simulink model "PMSM_controller"  (R2021b)
settings: Solver=VariableStepAuto  StartTime=0.0  StopTime=1  RelTol=1e-3
values from neighbouring files (symbols this model uses):
  J = 0.2    [Para_Trial.m]
  Tmax = 27    [Para_Trial.m]
  Ts = 2e-6    (= 2e-06)    [Para_Trial.m]
  Tsc = 5e-5    (= 5e-05)    [Para_Trial.m]
libraries: eePmsmFieldOrientedControl x1
settings Model: Creator=Patron  LastModifiedBy=Patron
settings SolverCC: ZeroCrossAlgorithm=Adaptive
settings DataIOCC: SaveOutput=off  SaveTime=off
settings DebuggingCC: IgnoredZcDiagnostic=none

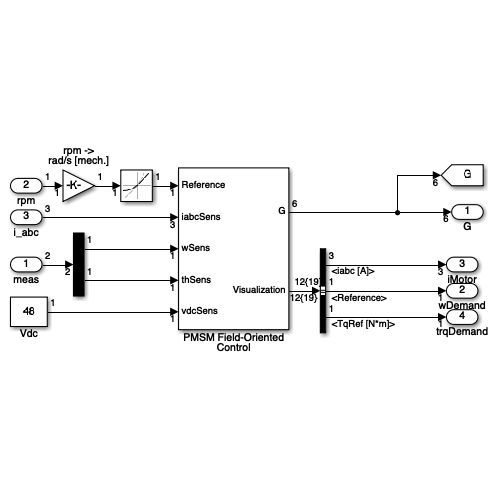
[thumbnail: Simulink's stored preview of the top-level diagram]
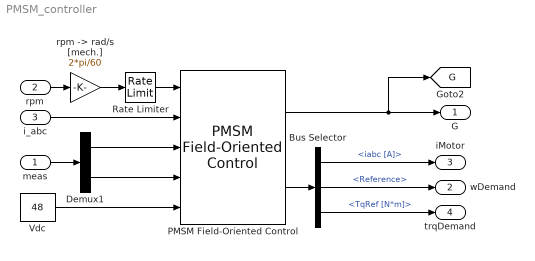
== system PMSM_controller ==
  meas : Inport  OutDataTypeStr=double  PortDimensions=2  SampleTime=[5.0000000000000002e-05,0]
  rpm : Inport  Port=2  OutDataTypeStr=double  PortDimensions=1  SampleTime=[5.0000000000000002e-05,0]
  i_abc : Inport  Port=3  OutDataTypeStr=double  PortDimensions=3  SampleTime=[5.0000000000000002e-05,0]
  Bus Selector : BusSelector  OutputSignals=iabc [A],Reference,TqRef [N*m]
  Demux1 : Demux  Outputs=2
  PMSM Field-Oriented Control : eePmsmFieldOrientedControl/PMSM Field-Oriented Control  winding_type=Wye-wound  CtrlMode=Torque control  Vnom=48  Pmax=Pmax  Tmax=Tmax*1.5  p=N  Vdc_on=10  Ts=Ts  Tsc=Tsc  CtrlType=PI control  Kp_w=60  Ki_w=300*2  Kv_w=1  Kaw_w=1000  RefType=Zero d-axis control  rpmVec=[0, 3000]  TqVec=[-100, 0, 100]  VdcVec=[300, 350]  PWMMode=SPWM: sinusoidal PWM  ModFactor=1  idMatrix=zeros(2,3,2)  iqMatrix=zeros(2,3,2)  psim=PM  Ld=0.00024  Lq=0.00029  Rs=0.01  AxisAlignment=Q-axis  Kp_id=0.1  Ki_id=10  Kaw_id=1000  Kp_iq=0.1  Ki_iq=10  Kaw_iq=1000  AxisPrio=Q-axis  ActZC=off  ActFF=on  ParamTypeFF=Constant parameters  LdFF=Ld  LqFF=Lq  psimFF=PM  idVect=[-200, 0, 200]  iqVect=[-200, 0, 200]  LdMatrix=0.0002 * ones(3, 3)  LqMatrix=0.0002 * ones(3, 3)  psimMatrix=0.04 * ones(3, 3)  CPWMMode=SPWM: sinusoidal PWM  fsw=fsw
      settings: SourceProductBaseCode=PS
  Rate Limiter : RateLimiter  RisingSlewLimit=Tmax/J  FallingSlewLimit=-Tmax/J  SampleTimeMode=inherited
  Vdc : Constant  Value=48  SampleTime=Tsc
  "rpm -> rad/s [mech.]" : Gain  Gain=2*pi/60
  G : Outport  OutDataTypeStr=double  PortDimensions=6  SampleTime=[1.9999999999999999e-06,0]  VectorParamsAs1DForOutWhenUnconnected=off
  wDemand : Outport  Port=2  OutDataTypeStr=double  PortDimensions=1
  iMotor : Outport  Port=3  OutDataTypeStr=double  PortDimensions=3
  trqDemand : Outport  Port=4  OutDataTypeStr=double  PortDimensions=1
  tag scope: G=global
  wires:
  PMSM Field-Oriented Control/1 -> [G], G/1
  Vdc/1 -> PMSM Field-Oriented Control/5
  PMSM Field-Oriented Control/2 -> Bus Selector/1
  i_abc/1 -> PMSM Field-Oriented Control/2
  meas/1 -> Demux1/1
  Demux1/1 -> PMSM Field-Oriented Control/3
  Demux1/2 -> PMSM Field-Oriented Control/4
  Bus Selector/1 -> iMotor/1  "<iabc [A]>"
  Bus Selector/2 -> wDemand/1  "<Reference>"
  Bus Selector/3 -> trqDemand/1  "<TqRef [N*m]>"
  rpm/1 -> "rpm -> rad/s [mech.]"/1
  Rate Limiter/1 -> PMSM Field-Oriented Control/1
  "rpm -> rad/s [mech.]"/1 -> Rate Limiter/1
